simulink model "MED2018_TireTest_Example"  (R2017b)
settings: Solver=ode1  StartTime=0.0  StopTime=10  FixedStep=0.01  RelTol=1e-3
libraries: simulink x1
settings Model: Creator=ashwin.ramanujam  LastModifiedBy=ashwin.ramanujam

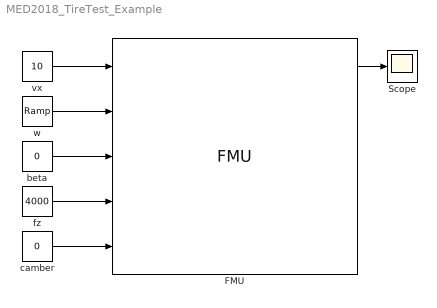
== system MED2018_TireTest_Example ==
  FMU : FMU  FMUName=MED2018_TireModel.fmu  FMUMode=CoSimulation  FMUSampleTime=-1  mask(Rimac.Vehicle.Wheels.TyreFMUContainer [Co-Simulation, v2.0]){}
      mask Display:
      | disp('Rimac.Vehicle.Wheels.TyreFMUContainer');
      | port_label('output',1,'Fx');
      | port_label('output',2,'Fy');
      | port_label('output',3,'Mz');
      | port_label('output',4,'r');
      | port_label('output',5,'Mx');
      | port_label('input',1,'vx');
      | port_label('input',2,'w');
      | port_label('input',3,'beta');
      | port_label('input',4,'Fz');
      | port_label('input',5,'camber');
  Scope : Scope
  beta : Constant  Value=0
  camber : Constant  Value=0
  fz : Constant  Value=4000
  vx : Constant  Value=10
  w : simulink/Sources/Ramp  slope=1  start=0  X0=25
  wires:
  vx/1 -> FMU/1
  w/1 -> FMU/2
  FMU/1 -> Scope/1
  beta/1 -> FMU/3
  fz/1 -> FMU/4
  camber/1 -> FMU/5
